simulink model "model_5"  (R2020b)
settings: Solver=VariableStepAuto  StartTime=0.0  StopTime=10.0  RelTol=1e-3
libraries: simulink x2
settings Model: Creator=Chetan  LastModifiedBy=Chetan

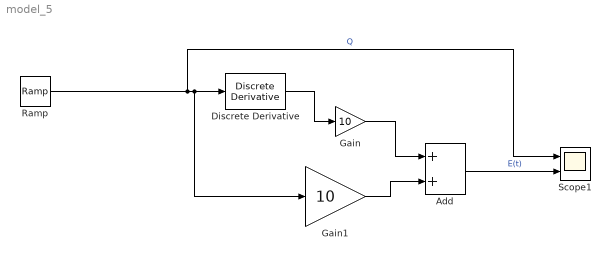
== system model_5 ==
  Add : Sum
  Discrete Derivative : simulink/Discrete/Discrete Derivative  gainval=1.0  ICPrevScaledInput=5  OutMin=[]  OutMax=[]  OutDataType=fixdt(1, 16)  OutScaling=2^-10  DoSatur=off
  Gain : Gain  Gain=10
  Gain1 : Gain  Gain=10
  Ramp : simulink/Sources/Ramp  slope=1  start=0  InitialOutput=0
  Scope1 : Scope  NumInputPorts=2
  wires:
  Ramp/1 -> Scope1/1, Discrete Derivative/1, Gain1/1  "Q"
  Discrete Derivative/1 -> Gain/1
  Gain/1 -> Add/1
  Gain1/1 -> Add/2
  Add/1 -> Scope1/2  "E(t)"
